simulink model "RL_vehicle_dynamic_model02"  (R2019b)
settings: Solver=ode45  StartTime=0.0  StopTime=60  RelTol=1e-3
model workspace (MAT data in the model file):
  kappar = [0 0 0 0 0 0 0 0 0 0 0 0 ... (4802 elements, 1x4802)]
  thetar = [0 0 0 0 0 0 0 0 0 0 0 0 ... (4802 elements, 1x4802)]
  xr = [0.0501253132832 0.100250626566 0.15037593985 0.200501253133 0.250626566416 0.300751879699 0.350877192982 0.401002506266 0.451127819549 0.501253132832 0.551378446115 0.601503759398 ... (4802 elements, 1x4802)]
  yr = [0 0 0 0 0 0 0 0 0 0 0 0 ... (4802 elements, 1x4802)]
libraries: simulink x3, rllib x1
(part 1 of 2)
settings Model: OrderedModelArguments=off  Creator=JHD  LastModifiedBy=JHD

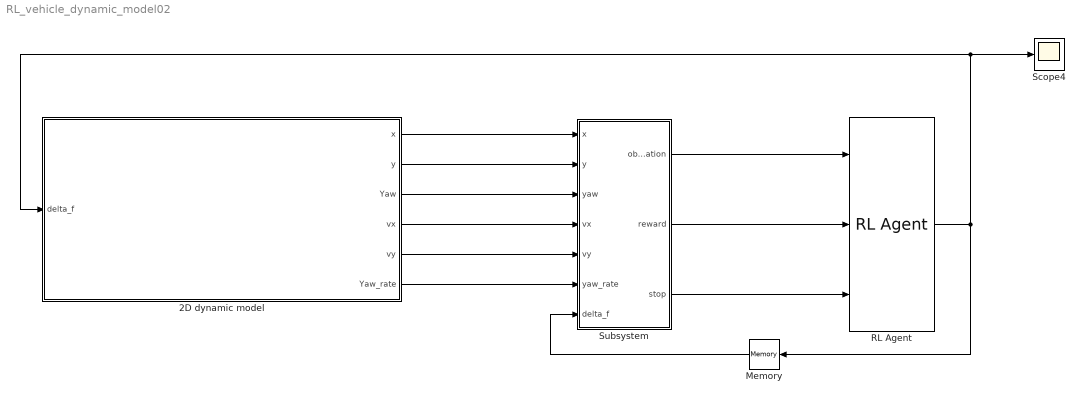
== system RL_vehicle_dynamic_model02 ==
  2D dynamic model : Subsystem
  Memory : Memory
  RL Agent : rllib/RL Agent  Agent=saved_agent  ProvideReward=on  ProvideIsDone=on  ProvideCumRwd=off  TreatAsDirectFeedthrough=on  CollectLoggedSignals=on  CollectModelStates=on
      settings: SourceProductName=Reinforcement Learning Toolbox
  Scope4 : Scope
  Subsystem : Subsystem
  wires:
  2D dynamic model/1(x) -> Subsystem/1(x)
  2D dynamic model/2(y) -> Subsystem/2(y)
  2D dynamic model/3(Yaw) -> Subsystem/3(yaw)
  2D dynamic model/4(vx) -> Subsystem/4(vx)
  2D dynamic model/5(vy) -> Subsystem/5(vy)
  2D dynamic model/6(Yaw_rate) -> Subsystem/6(yaw_rate)
  Subsystem/1(observation) -> RL Agent/1
  Subsystem/2(reward) -> RL Agent/2
  Subsystem/3(stop) -> RL Agent/3
  Memory/1 -> Subsystem/7(delta_f)
  RL Agent/1 -> Scope4/1, 2D dynamic model/1(delta_f), Memory/1
